simulink model "etc_mask1"  (R2024b)
settings: Solver=FixedStepAuto  StartTime=0.0  StopTime=10.0  FixedStep=0.01  RelTol=1e-3
values from neighbouring files (symbols this model uses):
  Ki = 2    [allParamValues.mat]
  Kp = 0.3    [allParamValues.mat]
  Ts = 0.01    [allParamValues.mat]
settings Model: Creator=trishkaya.harisunker  LastModifiedBy=trishkaya.harisunker

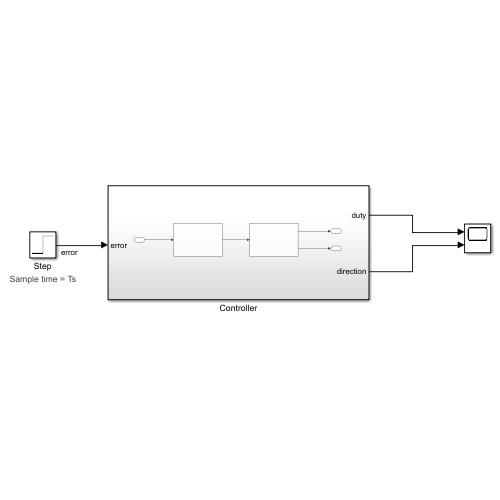
[thumbnail: Simulink's stored preview of the top-level diagram]
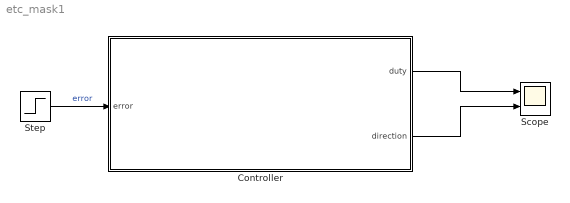
== system etc_mask1 ==
  Controller : Subsystem
  Scope : Scope  NumInputPorts=2
  Step : Step  SampleTime=Ts
      settings: AttributesFormatString=Sample time = %<SampleTime>
  wires:
  Step/1 -> Controller/1(error)  "error"
  Controller/2(direction) -> Scope/2
  Controller/1(duty) -> Scope/1

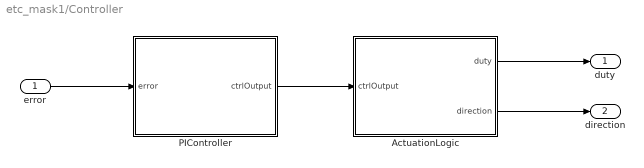
== system etc_mask1/Controller ==
  error : Inport
  ActuationLogic : Subsystem
  PIController : Subsystem
  duty : Outport
  direction : Outport  Port=2
  wires:
  ActuationLogic/1(duty) -> duty/1
  PIController/1(ctrlOutput) -> ActuationLogic/1(ctrlOutput)
  ActuationLogic/2(direction) -> direction/1
  error/1 -> PIController/1(error)

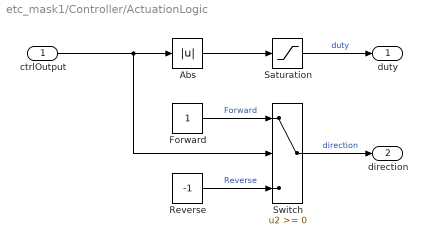
== system etc_mask1/Controller/ActuationLogic ==
  ctrlOutput : Inport
  Abs : Abs  SaturateOnIntegerOverflow=off
  Forward : Constant  OutDataTypeStr=double
  Reverse : Constant  Value=-1  OutDataTypeStr=double
  Saturation : Saturate  UpperLimit=1  LowerLimit=0
      settings: AttributesFormatString=%<LowerLimit> < duty < %<UpperLimit>
  Switch : Switch  SaturateOnIntegerOverflow=off  InputSameDT=off
      settings: AttributesFormatString=Criteria: %<Criteria>\nThreshold: %<Threshold>
  duty : Outport  VectorParamsAs1DForOutWhenUnconnected=off
  direction : Outport  Port=2  VectorParamsAs1DForOutWhenUnconnected=off
  wires:
  ctrlOutput/1 -> Abs/1, Switch/2
  Switch/1 -> direction/1  "direction"
  Abs/1 -> Saturation/1
  Reverse/1 -> Switch/3  "Reverse"
  Forward/1 -> Switch/1  "Forward"
  Saturation/1 -> duty/1  "duty"

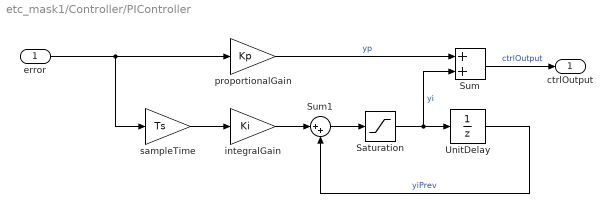
== system etc_mask1/Controller/PIController ==
  error : Inport
  Saturation : Saturate  UpperLimit=1  LowerLimit=-1
      settings: AttributesFormatString=Max: %<UpperLimit>\nMin: %<LowerLimit>
  Sum : Sum  InputSameDT=on  SaturateOnIntegerOverflow=on  OutDataTypeStr=Inherit: Same as first input
  Sum1 : Sum  Inputs=|++  InputSameDT=on  SaturateOnIntegerOverflow=on  OutDataTypeStr=Inherit: Same as first input
  UnitDelay : UnitDelay  SampleTime=Ts  HasFrameUpgradeWarning=on
      settings: AttributesFormatString=yi0 = %<X0>\nSample time = %<SampleTime>
  integralGain : Gain  Gain=Ki  SaturateOnIntegerOverflow=on  OutDataTypeStr=Inherit: Same as input  ParamDataTypeStr=Inherit: Same as input
  proportionalGain : Gain  Gain=Kp  SaturateOnIntegerOverflow=on  OutDataTypeStr=Inherit: Same as input  ParamDataTypeStr=Inherit: Same as input
  sampleTime : Gain  Gain=Ts  SaturateOnIntegerOverflow=on  OutDataTypeStr=Inherit: Same as input  ParamDataTypeStr=Inherit: Same as input
  ctrlOutput : Outport  VectorParamsAs1DForOutWhenUnconnected=off
  wires:
  Sum1/1 -> Saturation/1
  proportionalGain/1 -> Sum/1  "yp"
  Sum/1 -> ctrlOutput/1  "ctrlOutput"
  UnitDelay/1 -> Sum1/2  "yiPrev"
  Saturation/1 -> UnitDelay/1, Sum/2  "yi"
  integralGain/1 -> Sum1/1
  error/1 -> sampleTime/1, proportionalGain/1
  sampleTime/1 -> integralGain/1
